simulink model "ASLIPrun"  (R2015a)
settings: Solver=ode45  StartTime=0.0  StopTime=10.0  RelTol=1e-3
InitFcn:
  | ASLIPrun_params
values from neighbouring files (symbols this model uses):
  dt0 = -0.3325    [SLIPquad_params.m]
  dx0 = 0.4138    [SLIPquad_params.m]    (also in SLIPrun_params.m = 3; SLIPwalk_params.m = 2.5; smm_params.m = 5)
  dy0 = 0.1683    [SLIPquad_params.m]    (also in SLIPrun_params.m = -1; SLIPwalk_params.m = 0; smm_params.m = 0)
  g = 1    [SLIPquad_params.m]    (also in SLIPrun_params.m = 9.81; SLIPwalk_params.m = 9.81; smm_params.m = 9.81)
  J = 0.6    [SLIPquad_params.m]
  k = 20    [SLIPquad_params.m]    (also in SLIPrun_params.m = 23000; SLIPwalk_params.m = 10000; smm_params.m = 20000)
  L = sqrt( (u(3)-u(1))^2 + (u(4)-u(2))^2 )    [AnimSMR.m]    (also in SLIPquad_params.m = 0.5)
  l0 = 1    [SLIPquad_params.m]    (also in SLIPrun_params.m; SLIPwalk_params.m; smm_params.m)
  m = 1    [SLIPquad_params.m]    (also in SLIPrun_params.m = 70; SLIPwalk_params.m = 70; smm_params.m = 80)
  t0 = 0.056    [SLIPquad_params.m]
  x0 = []    [AnimQUAD.m]    (also in AnimQUAD2.m; AnimSMR.m; SLIPquad_params.m = 0; SLIPrun_params.m = -l*sin(theta_th))
  y0 = 1.0237    [SLIPquad_params.m]    (also in SLIPrun_params.m = sqrt(l^2 - x0^2); SLIPwalk_params.m = sqrt(l0^2 - x0^2); smm_params.m = 1)
undefined symbols (not defined in the file or in its folder): angle_attack
libraries: simulink_extras x1
settings Model: Creator=Joe  LastModifiedBy=Joe

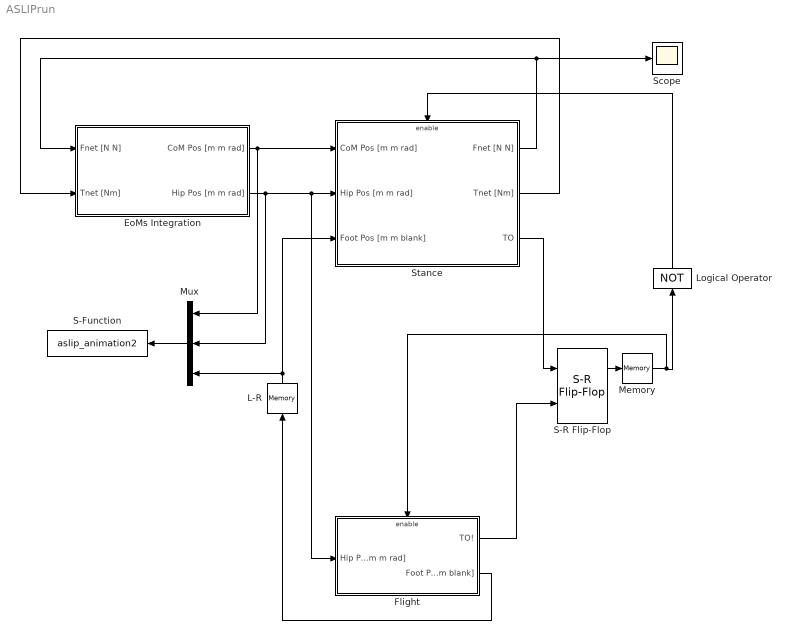
== system ASLIPrun ==
  EoMs Integration : Subsystem
  Flight : Subsystem
  L-R : Memory
  Logical Operator : Logic  Operator=NOT  AllPortsSameDT=off  OutDataTypeStr=boolean
  Memory : Memory
  Mux : Mux  Inputs=3
  S-Function : S-Function  FunctionName=aslip_animation2  Parameters=0.001
  S-R Flip-Flop : simulink_extras/Flip Flops/S-R Flip-Flop  initial_condition=0
  Scope : Scope
      settings: YMin=-3000  YMax=500
  Stance : Subsystem
  wires:
  EoMs Integration/2(Hip Pos [m m rad]) -> Mux/2, Flight/1(Hip Pos [m m rad]), Stance/2(Hip Pos [m m rad])
  EoMs Integration/1(CoM Pos [m m rad]) -> Mux/1, Stance/1("CoM Pos [m m rad] ")
  S-R Flip-Flop/1 -> Memory/1
  Stance/3(TO) -> S-R Flip-Flop/1
  Flight/1(TO!) -> S-R Flip-Flop/2
  Stance/2(Tnet [Nm]) -> EoMs Integration/2(Tnet [Nm])
  Memory/1 -> Logical Operator/1, Flight/Enable
  Logical Operator/1 -> Stance/Enable
  Flight/2(Foot Pos [m m blank]) -> L-R/1
  L-R/1 -> Stance/3(Foot Pos [m m blank]), Mux/3
  Mux/1 -> S-Function/1
  Stance/1(Fnet [N N]) -> EoMs Integration/1(Fnet [N N]), Scope/1

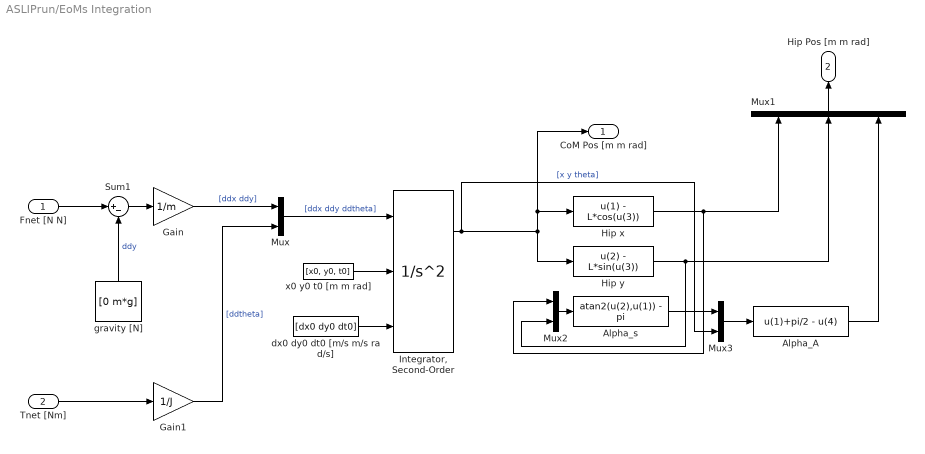
== system ASLIPrun/EoMs Integration ==
  Fnet [N N] : Inport
  Tnet [Nm] : Inport  Port=2
  Alpha_A : Fcn  Expr=u(1)+pi/2 - u(4)
  Alpha_s : Fcn  Expr=atan2(u(2),u(1)) - pi
  Gain : Gain  Gain=1/m
  Gain1 : Gain  Gain=1/J
  Hip x : Fcn  Expr=u(1) - L*cos(u(3))
  Hip y : Fcn  Expr=u(2) - L*sin(u(3))
  "Integrator, Second-Order" : SecondOrderIntegrator  ICSourceX=external  ICSourceDXDT=external
  Mux : Mux  Inputs=2
  Mux1 : Mux  Inputs=3
  Mux2 : Mux  Inputs=2
  Mux3 : Mux  Inputs=2
  Sum1 : Sum  Inputs=|+-
  dx0 dy0 dt0 [m/s m/s ra d/s] : Constant  Value=[dx0 dy0 dt0]
  gravity [N] : Constant  Value=[0 m*g]
  x0 y0 t0 [m m rad] : Constant  Value=[x0, y0, t0]
  CoM Pos [m m rad] : Outport
  Hip Pos [m m rad] : Outport  Port=2
  wires:
  "Integrator, Second-Order"/1 -> Mux3/2, CoM Pos [m m rad]/1, Hip x/1, Hip y/1  "[x y theta]"
  Sum1/1 -> Gain/1
  gravity [N]/1 -> Sum1/2  "ddy"
  x0 y0 t0 [m m rad]/1 -> "Integrator, Second-Order"/2
  Gain/1 -> Mux/1  "[ddx ddy]"
  Fnet [N N]/1 -> Sum1/1
  dx0 dy0 dt0 [m/s m/s ra d/s]/1 -> "Integrator, Second-Order"/3
  Mux/1 -> "Integrator, Second-Order"/1  "[ddx ddy ddtheta]"
  Gain1/1 -> Mux/2  "[ddtheta]"
  Tnet [Nm]/1 -> Gain1/1
  Hip x/1 -> Mux2/1, Mux1/1
  Hip y/1 -> Mux2/2, Mux1/2
  Mux1/1 -> Hip Pos [m m rad]/1
  Mux2/1 -> Alpha_s/1
  Mux3/1 -> Alpha_A/1
  Alpha_s/1 -> Mux3/1
  Alpha_A/1 -> Mux1/3

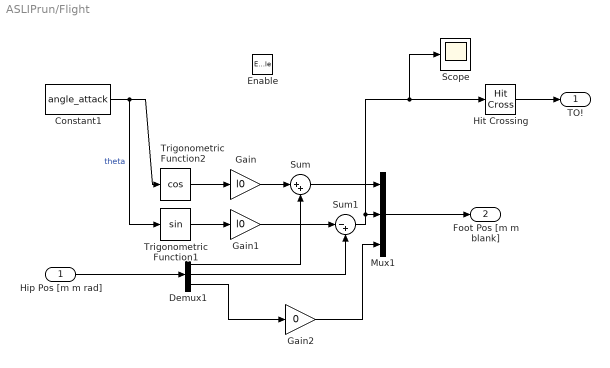
== system ASLIPrun/Flight ==
  Hip Pos [m m rad] : Inport
  Enable : EnablePort  StatesWhenEnabling=reset
  Constant1 : Constant  Value=angle_attack
  Demux1 : Demux  Outputs=3
  Gain : Gain  Gain=l0
  Gain1 : Gain  Gain=l0
  Gain2 : Gain  Gain=0
  Hit Crossing : HitCross  HitCrossingDirection=falling
  Mux1 : Mux  Inputs=3
  Scope : Scope
      settings: YMin=-0.025  YMax=0.175
  Sum : Sum  Inputs=|++
  Sum1 : Sum  Inputs=|-+
  Trigonometric Function1 : Trigonometry
  Trigonometric Function2 : Trigonometry  Operator=cos
  TO! : Outport  OutputWhenDisabled=reset  InitialOutput=[0]
  Foot Pos [m m blank] : Outport  Port=2  InitialOutput=[0 0 0]
  wires:
  Constant1/1 -> Trigonometric Function1/1, Trigonometric Function2/1  "theta"
  Trigonometric Function2/1 -> Gain/1
  Trigonometric Function1/1 -> Gain1/1
  Gain1/1 -> Sum1/1
  Gain/1 -> Sum/1
  Demux1/1 -> Sum/2
  Demux1/2 -> Sum1/2
  Sum1/1 -> Scope/1, Hit Crossing/1, Mux1/2
  Sum/1 -> Mux1/1
  Mux1/1 -> Foot Pos [m m blank]/1
  Hip Pos [m m rad]/1 -> Demux1/1
  Hit Crossing/1 -> TO!/1
  Gain2/1 -> Mux1/3
  Demux1/3 -> Gain2/1

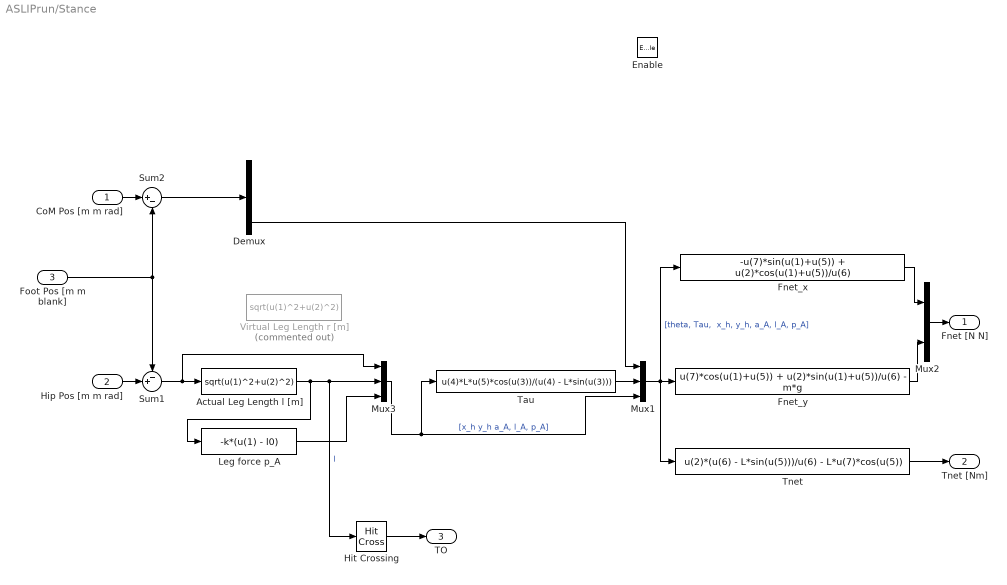
== system ASLIPrun/Stance ==
  "CoM Pos [m m rad] " : Inport
  Hip Pos [m m rad] : Inport  Port=2
  Foot Pos [m m blank] : Inport  Port=3
  Enable : EnablePort
  Actual Leg Length l [m] : Fcn  Expr=sqrt(u(1)^2+u(2)^2)
  Demux : Demux  Outputs=3
  Fnet_x : Fcn  Expr=-u(7)*sin(u(1)+u(5)) + u(2)*cos(u(1)+u(5))/u(6)
  Fnet_y : Fcn  Expr=u(7)*cos(u(1)+u(5)) + u(2)*sin(u(1)+u(5))/u(6) - m*g
  Hit Crossing : HitCross  HitCrossingOffset=l0  HitCrossingDirection=rising
  Leg force p_A : Fcn  Expr=-k*(u(1) - l0)
  Mux1 : Mux  Inputs=3
  Mux2 : Mux  Inputs=2
  Mux3 : Mux  Inputs=3
  Sum1 : Sum  Inputs=-+|
  Sum2 : Sum  Inputs=|+-
  Tau : Fcn  Expr=u(4)*L*u(5)*cos(u(3))/(u(4) - L*sin(u(3)))
  Tnet : Fcn  Expr=u(2)*(u(6) - L*sin(u(5)))/u(6) - L*u(7)*cos(u(5))
  Virtual Leg Length r [m] : Fcn  Commented=on  Expr=sqrt(u(1)^2+u(2)^2)
  Fnet [N N] : Outport  OutputWhenDisabled=reset  InitialOutput=[0,0]
  Tnet [Nm] : Outport  Port=2  OutputWhenDisabled=reset  InitialOutput=[0]
  TO : Outport  Port=3  OutputWhenDisabled=reset  InitialOutput=[0]
  wires:
  Leg force p_A/1 -> Mux3/3
  Mux3/1 -> Mux1/3, Tau/1  "[x_h y_h a_A, l_A, p_A]"
  Tau/1 -> Mux1/2
  Demux/3 -> Mux1/1
  Fnet_y/1 -> Mux2/2
  Fnet_x/1 -> Mux2/1
  Mux2/1 -> Fnet [N N]/1
  Tnet/1 -> Tnet [Nm]/1
  Actual Leg Length l [m]/1 -> Hit Crossing/1, Mux3/2, Leg force p_A/1  "l"
  Hit Crossing/1 -> TO/1
  Sum2/1 -> Demux/1
  "CoM Pos [m m rad] "/1 -> Sum2/1
  Sum1/1 -> Mux3/1, Actual Leg Length l [m]/1
  Hip Pos [m m rad]/1 -> Sum1/2
  Mux1/1 -> Tnet/1, Fnet_x/1, Fnet_y/1  "[theta, Tau,  x_h, y_h, a_A, l_A, p_A]"
  Foot Pos [m m blank]/1 -> Sum2/2, Sum1/1
